simulink model "farrow_filter"  (R2023a)
settings: Solver=VariableStepAuto  StartTime=0.0  StopTime=1024  RelTol=1e-3
undefined symbols (not defined in the file): S, vsva2197, xcvc1902
libraries: aieBasic x5, dspsrcs4 x1, vmcUtilities x1
settings Model: Creator=robg  LastModifiedBy=robg
settings DebuggingCC: ParameterPrecisionLossMsg=none

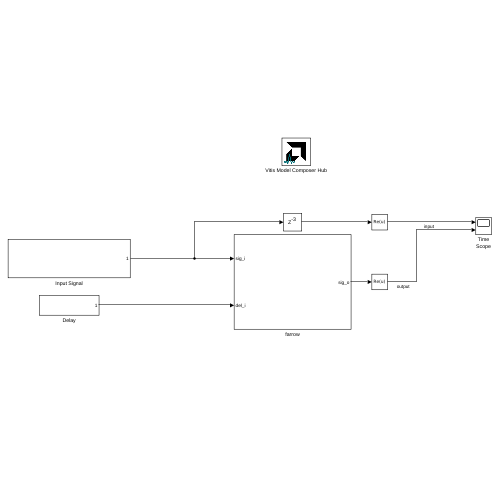
[thumbnail: Simulink's stored preview of the top-level diagram]
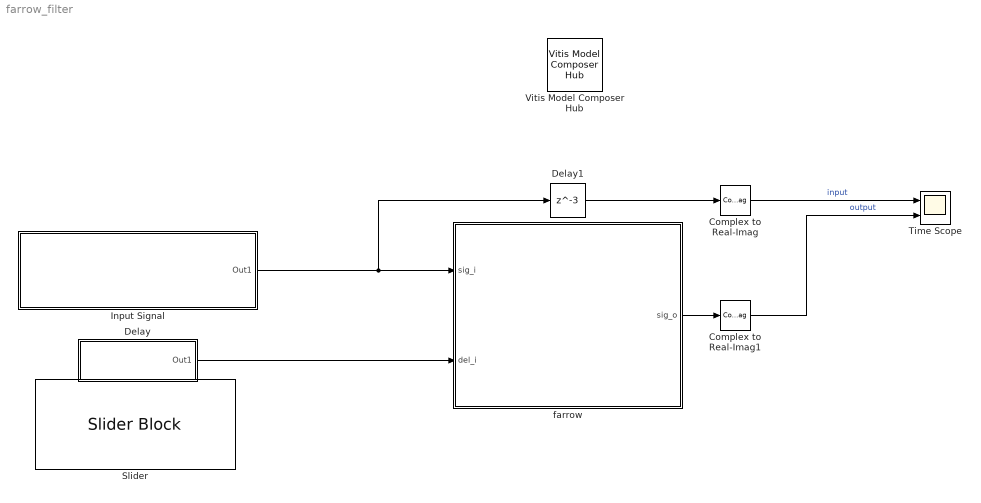
== system farrow_filter ==
  Complex to Real-Imag : ComplexToRealImag  Output=Real
  Complex to Real-Imag1 : ComplexToRealImag  Output=Real
  Delay : Subsystem
  Delay1 : Delay  DelayLength=3  InputProcessing=Columns as channels (frame based)
  Input Signal : Subsystem
  Slider : SliderBlock  LabelPosition=Hide  ScaleMin=-0.5  ScaleMax=0.5
  Time Scope : Scope  NumInputPorts=2
  Vitis Model Composer Hub : vmcUtilities/Vitis Model Composer Hub  Tag=genX  CodeGeneration=off  SubsystemName=farrow  CompilationType=HWCompilation  SubsystemType=AIENode  ExportTypeV2=Graph Code  StartColumn=1  NumberOfColumns=1  TargetDirectory=./code  exportDesign=off  analyzeDesign=off  validateDesignOnHw=on  ExportType=HW Code  IpVendor=xilinx.com  IpLibrary=hls  IpVersion=1.0  IpHWLanguage=Verilog  AieCompilerOptions={}  AieSimulatorOptions={}  CreateTestbench=off  TestbenchStackSize=10  RunRtlSim=off  RunCSim=off  RunAieSim=on  AieSimTimeout=50000  RunAieSimProfiling=off  LaunchVitisAnalyzer=off  PlotOutput=off  RunX86Sim=off  X86SimTimeout=10  GenHwImage=on  GenLibadfXo=off  GenHwValidationCode=off  PlatformType=Specify Platform  Platform=/proj/xbuilds/SWIP/2024.1_0522_2023/installs/lin64/Vitis/2024.1/base_platforms/xilinx_vck190_base_202410_1/xilinx_vck190_base_202410_1.xpfm  HwSystemType=Baremetal  HwValidationTarget=hw_emu  ProjDevice=Versal VCK190 Evaluation Platform (xcvc1902-vsva2197-2MP-e-S)  ProjDevicePart=xcvc1902-vsva2197-2MP-e-S  AIEType=AIE  SamplePeriod=-1  ClockFrequency=200  DataPathParallelism=1  xilinxfamily=versalaicore  part=xcvc1902  speed=-2MP-e-S  package=vsva2197  directory=./netlist  testbench=off  incr_netlist=off  synthesis_tool=Vivado  clock_wrapper=Clock Enables  dbl_ovrd=According to Block Masks  dcm_input_clock_period=10  sysclk_period=10  simulink_period=1  eval_field=0  IPInfoJsonString="{\"AIESubsystem\":{\"SubsystemName\":\"farrow\",\"TargetDirectory\":\"./code\",\"SubsystemDir\":\"./code/ip/farrow\"},\"SubsystemTag\":\"AIENode\"}"  LogFileName=/group/xcoswmktg2/robg/git/vmc_examples/Vitis_Model_Composer/Examples/AIENGINE/Farrow_Filter/code/model_composer.log  NThreads=4
  farrow : Subsystem
  wires:
  farrow/1(sig_o) -> Complex to Real-Imag1/1
  Complex to Real-Imag/1 -> Time Scope/1  "input"
  Complex to Real-Imag1/1 -> Time Scope/2  "output"
  Delay/1(Out1) -> farrow/2(del_i)
  Input Signal/1(Out1) -> Delay1/1, farrow/1(sig_i)
  Delay1/1 -> Complex to Real-Imag/1

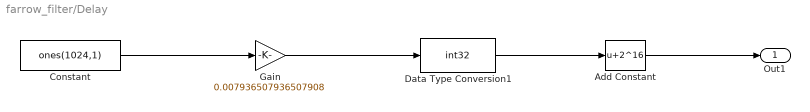
== system farrow_filter/Delay ==
  Add Constant : Bias  Bias=2^16  SaturateOnIntegerOverflow=off
  Constant : Constant  Value=ones(1024,1)  OutDataTypeStr=fixdt(1,16,14)  SampleTime=1024
  Data Type Conversion1 : DataTypeConversion  OutDataTypeStr=int32  ConvertRealWorld=Stored Integer (SI)  SaturateOnIntegerOverflow=off  RndMeth=Floor
  Gain : Gain  Gain=0.007936507936507908  OutDataTypeStr=Inherit: Same as input  ParamDataTypeStr=Inherit: Same as input
  Out1 : Outport
  wires:
  Gain/1 -> Data Type Conversion1/1
  Data Type Conversion1/1 -> Add Constant/1
  Add Constant/1 -> Out1/1
  Constant/1 -> Gain/1

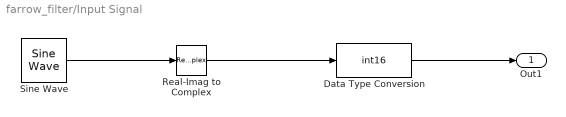
== system farrow_filter/Input Signal ==
  Data Type Conversion : DataTypeConversion  OutDataTypeStr=int16  SaturateOnIntegerOverflow=off  RndMeth=Floor
  Real-Imag to Complex : RealImagToComplex  Input=Real
  Sine Wave : dspsrcs4/Sine Wave  Amplitude=2^8  Frequency=1/32  Phase=0  SampleMode=Discrete  OutComplex=Real  CompMethod=Trigonometric fcn  TableSize=Speed  SampleTime=1  SamplesPerFrame=1024  ResetState=Restart at time zero  OutputFrames=off  dataType=double  wordLen=16  udDataType=sfix(16)  fracBitsMode=Best precision  numFracBits=15  OutDataTypeStr=double  LastOutDataTypeStr=double
  Out1 : Outport
  wires:
  Real-Imag to Complex/1 -> Data Type Conversion/1
  Sine Wave/1 -> Real-Imag to Complex/1
  Data Type Conversion/1 -> Out1/1

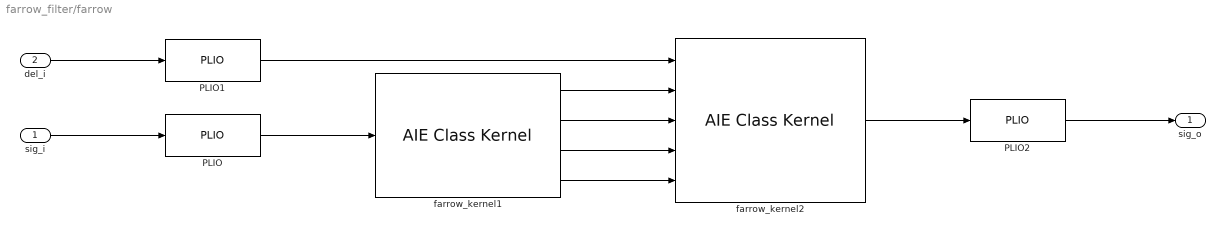
== system farrow_filter/farrow ==
  sig_i : Inport
  del_i : Inport  Port=2
  PLIO : aieBasic/PLIO  PlioWidth=64  PlioFreqSpec=off  PlioFreq=250  ColLocation=0  channel=0  blockJsonConstraints=[]  deprecateConstraints=0
  PLIO1 : aieBasic/PLIO  PlioWidth=64  PlioFreqSpec=off  PlioFreq=250  ColLocation=0  channel=0  blockJsonConstraints=[]  deprecateConstraints=0
  PLIO2 : aieBasic/PLIO  PlioWidth=64  PlioFreqSpec=off  PlioFreq=250  ColLocation=0  channel=0  blockJsonConstraints=[]  deprecateConstraints=0
  farrow_kernel1 : aieBasic/AIE Class Kernel  KernelAllAttrs=|  PortNames={'sig_i'; 'y3'; 'y2'; 'y1'; 'y0'}  PortSerializedTypes={'{Q2{R{Tadf::input_buffer{2{t{Scint16}}{t{Tadf::extents{1{t{}1024}}}}}}}}'; '{Q2{R{Tadf::output_buffer{2{t{Scint16}}{t{Tadf::extents{1{t{}1024}}}}}}}}'; '{Q2{R{Tadf::output_buffer{2{t{Scint16}}{t{Tadf::extents{1{t{}1024}}}}}}}}'; '{Q2{R{Tadf::output_buffer{2{t{Scint16}}{t{Tadf::extents{1{t{}1024}}}}}}}}'; '{Q2{R{Tadf::output_buffer{2{t{Scint16}}{t{Tadf::extents{1{t{}1024}}}}}}}}'}  PortWindowSizes={1.024000000000000000e+03; 1.024000000000000000e+03; 1.024000000000000000e+03; 1.024000000000000000e+03; 1.024000000000000000e+03}  PortWindowMargins={0.000000000000000000e+00; 0.000000000000000000e+00; 0.000000000000000000e+00; 0.000000000000000000e+00; 0.000000000000000000e+00}  PortSynchronicities={'sync', 'sync', 'sync', 'sync', 'sync'}  PortSignalSizes={0.000000000000000000e+00; 0.000000000000000000e+00; 0.000000000000000000e+00; 0.000000000000000000e+00; 0.000000000000000000e+00}  ClassTemplateSpecKind=none  ClassTemplateParamNames={}  ClassTemplateParamKinds={}  ClassTemplateParamTypes={}  ClassTemplateParamValues={}  ClassCtorParamNames={}  ClassCtorParamSerializedTypes={}  ClassCtorParamValues={}  ClassIndex=1  ClassCtorIndex=0  ClassTabVisible=on  ClassTemplateParamsVisible=off  ClassCtorDeclVisible=off  ClassCtorParamsVisible=off  FunctionTabVisible=on  FunctionDecl=|  PortAttrs={ 'input', 'sig_i', 'adf::input_buffer< cint16, adf::extents< 1024 > > & restrict', '1024', '0', 'sync', ''; 'output', 'y3', 'adf::output_buffer< cint16, adf::extents< 1024 > > & restrict', '1024', '', 'sync', ''; 'output', 'y2', 'adf::output_buffer< cint16, adf::extents< 1024 > > & restrict', '1024', '', 'sync', ''; 'output', 'y1', 'adf::output_buffer< cint16, adf::extents< 1024 > > & restrict', '1024', '', 'sync', ''; 'output', 'y0', 'adf::output_buffer< cint16, adf::extents< 1024 > > & restrict', '1024', '', 'sync', '' }  PortAttrsEnables={'off', 'off', 'off', 'off', 'off', 'off', 'off';'off', 'off', 'off', 'off', 'off', 'off', 'off';'off', 'off', 'off', 'off', 'off', 'off', 'off';'off', 'off', 'off', 'off', 'off', 'off', 'off';'off', 'off', 'off', 'off', 'off', 'off', 'off'}  SampleTime=-1  ClassDeclTypeOptions=C[1 1]@t21@class farrow_kernel1;  ClassDecl=class farrow_kernel1;  ClassTemplateParams={}  ClassTemplateParamsEnables={}  ClassCtorDeclTypeOptions=C[1 1]@t7@<empty>  ClassCtorDecl=<empty>  ClassCtorParams={}  KernelHeaderFile=aie/farrow_kernel1.h  KernelClassName=farrow_kernel1  KernelFunction=run  KernelSourceFile=aie/farrow_kernel1.cpp  KernelSearchPaths={}  PreProcOptions={}  blockJsonConstraints=[]
      KernelAllAttrs=|
      | s[12;12;9;9;19;14;21;23;21;23;24;21;15;17;12;24;26;26;26;27;28;9;21;23;23;23;24;25;14;19;19;29]@FunctionNameDeclFileNamePortNamesPortTypesPortSerializedTypesPortDirectionsPortWindowSizeEnablesPortWindowMarginEnablesPortBufferSizeEnablesPortBufferMarginEnablesPortSynchronicityEnablesPortSignalSizeEnablesPortBufferSizesPortBufferMarginsFunctionDeclFunctionTemplateSpecKindFunctionTemplateParamNamesFunctionTemplateParamKindsFunctionTemplateParamTypesFunctionTemplateParamValuesFunctionTemplateParamEnablesClassDeclClassTemplateSpecKindClassTemplateParamNamesClassTemplateParamKindsClassTemplateParamTypesClassTemplateParamValuesClassTemplateParamEnablesClassCtorDeclsClassCtorParamNamesClassCtorParamTypesClassCtorParamSerializedTypes[1 1]@C[32 1]@t3@runt26@../../aie/farrow_kernel1.hC[5 1]@t5@sig_it2@y3t2@y2t2@y1t2@y0C[5 1]@t60@adf::input_buffer< cint16, adf::extents< 1024 > > & restrictt61@adf::output_buffer< cint16, adf::extents< 1024 > > & restrictt61@adf::output_buffer< cint16, adf::extents< 1024 > > & restrictt61@adf::output_buffer< cint16, adf::extents< 1024 > > & restrictt61@adf::output_buffer< cint16, adf::extents< 1024 > > & restrictC[5 1]@t72@{Q2{R{Tadf::input_buffer{2{t{Scint16}}{t{Tadf::extents{1{t{}1024}}}}}}}}t73@{Q2{R{Tadf::output_buffer{2{t{Scint16}}{t{Tadf::extents{1{t{}1024}}}}}}}}t73@{Q2{R{Tadf::output_buffer{2{t{Scint16}}{t{Tadf::extents{1{t{}1024}}}}}}}}t73@{Q2{R{Tadf::output_buffer{2{t{Scint16}}{t{Tadf::extents{1{t{}1024}}}}}}}}t73@{Q2{R{Tadf::output_buffer{2{t{Scint16}}{t{Tadf::extents{1{t{}1024}}}}}}}}C[5 1]@t5@inputt6@outputt6@outputt6@outputt6@outputC[5 1]@l1@l1@l1@l1@l1@C[5 1]@l1@l0@l0@l0@l0@C[5 1]@l1@l1@l1@l1@l1@C[5 1]@l0@l0@l0@l0@l0@C[5 1]@l1@l1@l1@l1@l1@C[5 1]@l0@l0@l0@l0@l0@C[5 1]@t4@1024t4@1024t4@1024t4@1024t4@1024C[5 1]@nnnnnt357@void farrow_kernel1::
      | run(adf::input_buffer< cint16, adf::extents< 1024 > > & restrict sig_i, adf::output_buffer< cint16, adf::extents< 1024 > > & restrict y3, adf::output_buffer< cint16, adf::extents< 1024 > > & restrict y2, adf::output_buffer< cint16, adf::extents< 1024 > > & restrict y1, adf::output_buffer< cint16, adf::extents< 1024 > > & restrict y0)t4@nonee[0 1]@e[0 1]@e[0 1]@e[0 1]@e[0 1]@t21@class farrow_kernel1;t4@nonee[0 1]@e[0 1]@e[0 1]@e[0 1]@e[0 1]@e[0 1]@e[0 1]@e[0 1]@e[0 1]@
      FunctionDecl=|
      | void farrow_kernel1::
      | run(adf::input_buffer< cint16, adf::extents< 1024 > > & restrict sig_i, adf::output_buffer< cint16, adf::extents< 1024 > > & restrict y3, adf::output_buffer< cint16, adf::extents< 1024 > > & restrict y2, adf::output_buffer< cint16, adf::extents< 1024 > > & restrict y1, adf::output_buffer< cint16, adf::extents< 1024 > > & restrict y0)
  farrow_kernel2 : aieBasic/AIE Class Kernel  KernelAllAttrs=|  PortNames={'del_i'; 'y3'; 'y2'; 'y1'; 'y0'; 'sig_o'}  PortSerializedTypes={'{Q2{R{Tadf::input_buffer{2{t{Bi32}}{t{Tadf::extents{1{t{}1024}}}}}}}}'; '{Q2{R{Tadf::input_buffer{2{t{Scint16}}{t{Tadf::extents{1{t{}1024}}}}}}}}'; '{Q2{R{Tadf::input_buffer{2{t{Scint16}}{t{Tadf::extents{1{t{}1024}}}}}}}}'; '{Q2{R{Tadf::input_buffer{2{t{Scint16}}{t{Tadf::extents{1{t{}1024}}}}}}}}'; '{Q2{R{Tadf::input_buffer{2{t{Scint16}}{t{Tadf::extents{1{t{}1024}}}}}}}}'; '{Q2{R{Tadf::output_buffer{2{t{Scint16}}{t{Tadf::extents{1{t{}1024}}}}}}}}'}  PortWindowSizes={1.024000000000000000e+03; 1.024000000000000000e+03; 1.024000000000000000e+03; 1.024000000000000000e+03; 1.024000000000000000e+03; 1.024000000000000000e+03}  PortWindowMargins={0.000000000000000000e+00; 0.000000000000000000e+00; 0.000000000000000000e+00; 0.000000000000000000e+00; 0.000000000000000000e+00; 0.000000000000000000e+00}  PortSynchronicities={'sync', 'sync', 'sync', 'sync', 'sync', 'sync'}  PortSignalSizes={0.000000000000000000e+00; 0.000000000000000000e+00; 0.000000000000000000e+00; 0.000000000000000000e+00; 0.000000000000000000e+00; 0.000000000000000000e+00}  ClassTemplateSpecKind=none  ClassTemplateParamNames={}  ClassTemplateParamKinds={}  ClassTemplateParamTypes={}  ClassTemplateParamValues={}  ClassCtorParamNames={}  ClassCtorParamSerializedTypes={}  ClassCtorParamValues={}  ClassIndex=1  ClassCtorIndex=0  ClassTabVisible=on  ClassTemplateParamsVisible=off  ClassCtorDeclVisible=off  ClassCtorParamsVisible=off  FunctionTabVisible=on  FunctionDecl=|  PortAttrs={ 'input', 'del_i', 'adf::input_buffer< int32, adf::extents< 1024 > > & restrict', '1024', '0', 'sync', ''; 'input', 'y3', 'adf::input_buffer< cint16, adf::extents< 1024 > > & restrict', '1024', '0', 'sync', ''; 'input', 'y2', 'adf::input_buffer< cint16, adf::extents< 1024 > > & restrict', '1024', '0', 'sync', ''; 'input', 'y1', 'adf::input_buffer< cint16, adf::extents< 1024 > > & restrict', '1024', '0', 'sync', ''; 'input', 'y0', 'adf::input_buffer< cint16, adf::extents< 1024 > > & restrict', '1024', '0', 'sync', ''; 'output', 'sig_o', 'adf::output_buffer< cint16, adf::extents< 1024 > > & restrict', '1024', '', 'sync', '' }  PortAttrsEnables={'off', 'off', 'off', 'off', 'off', 'off', 'off';'off', 'off', 'off', 'off', 'off', 'off', 'off';'off', 'off', 'off', 'off', 'off', 'off', 'off';'off', 'off', 'off', 'off', 'off', 'off', 'off';'off', 'off', 'off', 'off', 'off', 'off', 'off';'off', 'off', 'off', 'off', 'off', 'off', 'off'}  SampleTime=-1  ClassDeclTypeOptions=C[1 1]@t21@class farrow_kernel2;  ClassDecl=class farrow_kernel2;  ClassTemplateParams={}  ClassTemplateParamsEnables={}  ClassCtorDeclTypeOptions=C[1 1]@t7@<empty>  ClassCtorDecl=<empty>  ClassCtorParams={}  KernelHeaderFile=aie/farrow_kernel2.h  KernelClassName=farrow_kernel2  KernelFunction=run  KernelSourceFile=aie/farrow_kernel2.cpp  KernelSearchPaths={}  PreProcOptions={}  blockJsonConstraints=[]
      KernelAllAttrs=|
      | s[12;12;9;9;19;14;21;23;21;23;24;21;15;17;12;24;26;26;26;27;28;9;21;23;23;23;24;25;14;19;19;29]@FunctionNameDeclFileNamePortNamesPortTypesPortSerializedTypesPortDirectionsPortWindowSizeEnablesPortWindowMarginEnablesPortBufferSizeEnablesPortBufferMarginEnablesPortSynchronicityEnablesPortSignalSizeEnablesPortBufferSizesPortBufferMarginsFunctionDeclFunctionTemplateSpecKindFunctionTemplateParamNamesFunctionTemplateParamKindsFunctionTemplateParamTypesFunctionTemplateParamValuesFunctionTemplateParamEnablesClassDeclClassTemplateSpecKindClassTemplateParamNamesClassTemplateParamKindsClassTemplateParamTypesClassTemplateParamValuesClassTemplateParamEnablesClassCtorDeclsClassCtorParamNamesClassCtorParamTypesClassCtorParamSerializedTypes[1 1]@C[32 1]@t3@runt26@../../aie/farrow_kernel2.hC[6 1]@t5@del_it2@y3t2@y2t2@y1t2@y0t5@sig_oC[6 1]@t59@adf::input_buffer< int32, adf::extents< 1024 > > & restrictt60@adf::input_buffer< cint16, adf::extents< 1024 > > & restrictt60@adf::input_buffer< cint16, adf::extents< 1024 > > & restrictt60@adf::input_buffer< cint16, adf::extents< 1024 > > & restrictt60@adf::input_buffer< cint16, adf::extents< 1024 > > & restrictt61@adf::output_buffer< cint16, adf::extents< 1024 > > & restrictC[6 1]@t69@{Q2{R{Tadf::input_buffer{2{t{Bi32}}{t{Tadf::extents{1{t{}1024}}}}}}}}t72@{Q2{R{Tadf::input_buffer{2{t{Scint16}}{t{Tadf::extents{1{t{}1024}}}}}}}}t72@{Q2{R{Tadf::input_buffer{2{t{Scint16}}{t{Tadf::extents{1{t{}1024}}}}}}}}t72@{Q2{R{Tadf::input_buffer{2{t{Scint16}}{t{Tadf::extents{1{t{}1024}}}}}}}}t72@{Q2{R{Tadf::input_buffer{2{t{Scint16}}{t{Tadf::extents{1{t{}1024}}}}}}}}t73@{Q2{R{Tadf::output_buffer{2{t{Scint16}}{t{Tadf::extents{1{t{}1024}}}}}}}}C[6 1]@t5@inputt5@inputt5@inputt5@inputt5@inputt6@outputC[6 1]@l1@l1@l1@l1@l1@l1@C[6 1]@l1@l1@l1@l1@l1@l0@C[6 1]@l1@l1@l1@l1@l1@l1@C[6 1]@l0@l0@l0@l0@l0@l0@C[6 1]@l1@l1@l1@l1@l1@l1@C[6 1]@l0@l0@l0@l0@l0@l0@C[6 1]@t4@1024t4@1024t4@1024t4@1024t4@1024t4@1024C[6 1]@nnnnnnt421@void farrow_kernel2::
      | run(adf::input_buffer< int32, adf::extents< 1024 > > & restrict del_i, adf::input_buffer< cint16, adf::extents< 1024 > > & restrict y3, adf::input_buffer< cint16, adf::extents< 1024 > > & restrict y2, adf::input_buffer< cint16, adf::extents< 1024 > > & restrict y1, adf::input_buffer< cint16, adf::extents< 1024 > > & restrict y0, adf::output_buffer< cint16, adf::extents< 1024 > > & restrict sig_o)t4@nonee[0 1]@e[0 1]@e[0 1]@e[0 1]@e[0 1]@t21@class farrow_kernel2;t4@nonee[0 1]@e[0 1]@e[0 1]@e[0 1]@e[0 1]@e[0 1]@e[0 1]@e[0 1]@e[0 1]@
      FunctionDecl=|
      | void farrow_kernel2::
      | run(adf::input_buffer< int32, adf::extents< 1024 > > & restrict del_i, adf::input_buffer< cint16, adf::extents< 1024 > > & restrict y3, adf::input_buffer< cint16, adf::extents< 1024 > > & restrict y2, adf::input_buffer< cint16, adf::extents< 1024 > > & restrict y1, adf::input_buffer< cint16, adf::extents< 1024 > > & restrict y0, adf::output_buffer< cint16, adf::extents< 1024 > > & restrict sig_o)
  sig_o : Outport
  wires:
  PLIO/1 -> farrow_kernel1/1
  PLIO1/1 -> farrow_kernel2/1
  farrow_kernel1/2 -> farrow_kernel2/3
  del_i/1 -> PLIO1/1
  farrow_kernel1/3 -> farrow_kernel2/4
  sig_i/1 -> PLIO/1
  farrow_kernel1/1 -> farrow_kernel2/2
  PLIO2/1 -> sig_o/1
  farrow_kernel2/1 -> PLIO2/1
  farrow_kernel1/4 -> farrow_kernel2/5
